simulink model "WDS2"  (R2022b)
settings: Solver=VariableStepAuto  StartTime=0.0  StopTime=86400  RelTol=0.034
libraries: sh_lib x46, nesl_utility x16, fl_lib x12, SignalEditorBlockLib x3
(part 1 of 2)
settings Model: Creator=philip  LastModifiedBy=philip
settings SolverCC: MaxConsecutiveMinStep=2

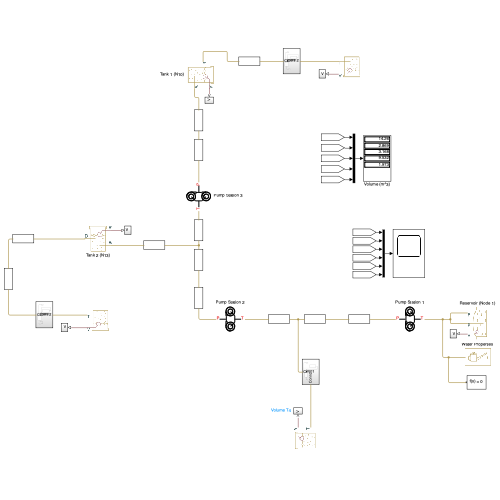
[thumbnail: Simulink's stored preview of the top-level diagram]
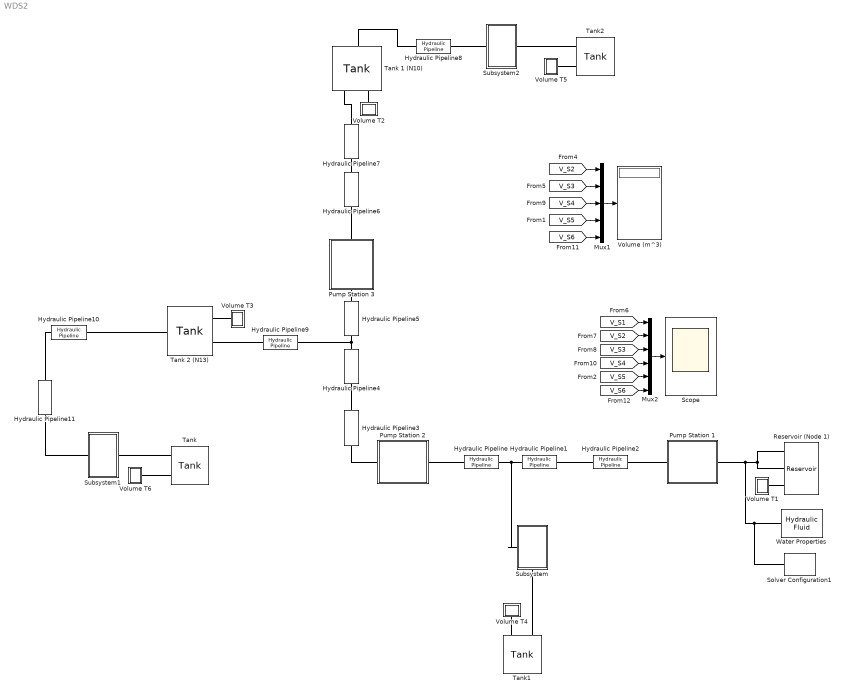
== system WDS2 ==
  Hydraulic Pipeline{,1..11} (12 alike) : sh_lib/Pipelines/Hydraulic Pipeline  cs_type=foundation.enum.pipeCrossSection.circular  d_in=0.01 m  area=1e-4 m^2  D_h=1.12e-2 m  s_factor=64  length=5 m  length_ad=1 m  roughness=15e-6 m  Re_lam=2000  Re_turb=4000  wall_type=foundation.enum.chamber_spec.rigid  pr_r_coef=2e-12 m/Pa  time_const=0.01 s  k_sh=1.4  initial_pressure=0 Pa
      settings: InternalSimscapePortConfiguration="{\"Bottom\":[],\"Left\":[{\"id\":\"A\",\"label\":\"A\",\"type\":\"foundation.hydraulic.hydraulic\"}],\"Right\":[{\"id\":\"B\",\"label\":\"B\",\"type\":\"foundation.hydraulic.hydraulic\"}],\"Top\":[]}"
  Mux1 : Mux  Inputs=5
  Mux2 : Mux  Inputs=6
  Pump Station 1 : Subsystem  Tag=PublishSubsystem
      mask Display:
      | plot(sin(0:0.5:4.5*pi)*0.9, cos(0:0.5:4.5*pi)*0.9+1.5)
      | plot(sin(0:0.5:4.5*pi)*0.5, cos(0:0.5:4.5*pi)*0.5+1.5)
      | plot(sin(0:0.5:4.5*pi)*0.9, cos(0:0.5:4.5*pi)*0.9-1.5)
      | plot(sin(0:0.5:4.5*pi)*0.5, cos(0:0.5:4.5*pi)*0.5-1.5)
      | 
      | plot([0 -0.9],[1.5 1.5-0.9])
      | plot([0 -0.9],[1.5 1.5-0.9]*-1)
      | 
      | plot([0.45 0.45 0.325 0.325]*2,[1.5 1.5-1.0 1.5-1.0 1.5-0.55])
      | plot([0.45 0.45 0.325 0.325]*2,[1.5 1.5-0.9 1.5-0.9 1.5-0.55]*-1)
      | 
      | plot([2.2 0.95]*-1,[0 0])
      | plot([2.2 0.95],[0 0])
      | 
      | plot([0.95 0.95]*-1,[-0.6 0.6])
      | plot([0.8 0.8],[-0.55 0.55])
      | 
      | 
      | color('white');plot(-3,-2.5);plot(3,2.5);
      | color('red');
      | port_label('LConn',1,'T');
      | port_label('RConn',1,'P');
  Pump Station 2 : Subsystem  Tag=PublishSubsystem
      mask Display:
      | plot(sin(0:0.5:4.5*pi)*0.9, cos(0:0.5:4.5*pi)*0.9+1.5)
      | plot(sin(0:0.5:4.5*pi)*0.5, cos(0:0.5:4.5*pi)*0.5+1.5)
      | plot(sin(0:0.5:4.5*pi)*0.9, cos(0:0.5:4.5*pi)*0.9-1.5)
      | plot(sin(0:0.5:4.5*pi)*0.5, cos(0:0.5:4.5*pi)*0.5-1.5)
      | 
      | plot([0 -0.9],[1.5 1.5-0.9])
      | plot([0 -0.9],[1.5 1.5-0.9]*-1)
      | 
      | plot([0.45 0.45 0.325 0.325]*2,[1.5 1.5-1.0 1.5-1.0 1.5-0.55])
      | plot([0.45 0.45 0.325 0.325]*2,[1.5 1.5-0.9 1.5-0.9 1.5-0.55]*-1)
      | 
      | plot([2.2 0.95]*-1,[0 0])
      | plot([2.2 0.95],[0 0])
      | 
      | plot([0.95 0.95]*-1,[-0.6 0.6])
      | plot([0.8 0.8],[-0.55 0.55])
      | 
      | 
      | color('white');plot(-3,-2.5);plot(3,2.5);
      | color('red');
      | port_label('LConn',1,'T');
      | port_label('RConn',1,'P');
  Pump Station 3 : Subsystem  Tag=PublishSubsystem
      mask Display:
      | plot(sin(0:0.5:4.5*pi)*0.9, cos(0:0.5:4.5*pi)*0.9+1.5)
      | plot(sin(0:0.5:4.5*pi)*0.5, cos(0:0.5:4.5*pi)*0.5+1.5)
      | plot(sin(0:0.5:4.5*pi)*0.9, cos(0:0.5:4.5*pi)*0.9-1.5)
      | plot(sin(0:0.5:4.5*pi)*0.5, cos(0:0.5:4.5*pi)*0.5-1.5)
      | 
      | plot([0 -0.9],[1.5 1.5-0.9])
      | plot([0 -0.9],[1.5 1.5-0.9]*-1)
      | 
      | plot([0.45 0.45 0.325 0.325]*2,[1.5 1.5-1.0 1.5-1.0 1.5-0.55])
      | plot([0.45 0.45 0.325 0.325]*2,[1.5 1.5-0.9 1.5-0.9 1.5-0.55]*-1)
      | 
      | plot([2.2 0.95]*-1,[0 0])
      | plot([2.2 0.95],[0 0])
      | 
      | plot([0.95 0.95]*-1,[-0.6 0.6])
      | plot([0.8 0.8],[-0.55 0.55])
      | 
      | 
      | color('white');plot(-3,-2.5);plot(3,2.5);
      | color('red');
      | port_label('LConn',1,'T');
      | port_label('RConn',1,'P');
  Reservoir (Node 1) : sh_lib/Hydraulic Utilities/Reservoir  press=0 Pa  init_volume=40 m^3  ret_diam=0.01 m  loss_coeff=1
      settings: InternalSimscapePortConfiguration="{\"Bottom\":[],\"Left\":[{\"id\":\"V\",\"label\":\"V\",\"type\":\"output\"},{\"id\":\"P\",\"label\":\"P\",\"type\":\"foundation.hydraulic.hydraulic\"},{\"id\":\"R\",\"label\":\"R\",\"type\":\"foundation.hydraulic.hydraulic\"}],\"Right\":[],\"Top\":[]}"
  Scope : Scope
  Solver Configuration1 : nesl_utility/Solver Configuration  PhysicalDomain=network_engine_domain  SubClassName=solver  LeftPortType=input  RightPortType=generic  Tones=[]  Harmonics=[]  SimulateNoise=off  Profile=off  UseLocalSampling=off  EnableSwitchedLinearOptims=on  FrequencyDomain=off  UseCCode=off  RelTol=0.001  AbsTol=1e-06  MinStep=1e-09  ToWorkspace=off  RevertToSquareIcSolve=off  NumHomotopyIterations=100  PhasorMode=off  PhasorModeNumHarmonics=1  ConsistencySolver=NEWTON_XTOL_AFTER_FTOL  IndexReductionMethod=DerivativeReplacement  DoDC=off  ResidualTolerance=1e-9  ConsistencyTolSource=GLOBAL  ConsistencyAbsTol=0.001  ConsistencyRelTol=0.001  ConsistencyTolFactor=0.034  UseLocalSolver=off  LocalSolverChoice=NE_BACKWARD_EULER_ADVANCER  ResolveIndetEquations=on  FunctionEvalNumThread=1  LocalSolverSampleTime=.001  DoFixedCost=off  MaxNonlinIter=3  MaxModeIter=2  ComputeImpulses=off  ImpulseIterations=2  LinearAlgebra=auto  LinearAlgebraNumThread=0  EquationFormulation=NE_TIME_EF  DelaysMemoryBudget=1024  AutomaticFiltering=on  FilteringTimeConstant=0.001  PartitionStorageMethod=AS_NEEDED  PartitionMemoryBudget=1024  PartitionMethod=FAST
  Subsystem : Subsystem
      settings: PortSchema="{\"entries\":[{\"content\":{\"sides\":[{\"content\":{\"connectorIds\":[\"LConn1\"]},\"type\":\"ConnectorPlacement.EquallySpacedRectSide\",\"uuid\":\"c5da6f35-8fa4-48b7-8a4a-4ae9db04ca9d\"},{\"content\":{\"connectorIds\":[],\"side\":\"RIGHT\"},\"type\":\"ConnectorPlacement.EquallySpacedRectSide\",\"uuid\":\"484dc1ab-2dc7-464f-80da-36af203a6e69\"},{\"content\":{\"connectorIds\":[],\"side\":\"TOP\"},\"type\":\"ConnectorPlacement.EquallySpacedRectSide\",\"uuid\":\"15bf6548-86e0-4373-a220-3fe0e1067d73\"},{\"content\":{\"connectorIds\":[\"RConn1\"],\"side\":\"BOTTOM\"},\"type\":\"ConnectorPlacement.EquallySpacedRectSide\",\"uuid\":\"b94051b1-e6bf-4793-98e6-5d6956093d36\"}]},\"type\":\"ConnectorPlacement.EquallySpacedConnector\",\"uuid\":\"b1159124-f196-4e4e-b402-5d78480e647c\"}],\"packageUris\":[\"http://schema.mathworks.com/mf0/Connector/R2020b\"],\"version\":\"1.0\"}"
  Subsystem1 : Subsystem
  Subsystem2 : Subsystem
  Tank : sh_lib/Low-Pressure Blocks/Tank  press=0 Pa  level_spec=1  tank_area=0.8 m^2  fluid_volume_tab=[0, .0028, .0065, .0114, .0176, .0252, .0344, .0436, .0512, .0574, .0623, .066, .0688, .0707, .072, .0727] m^3  fluid_level_tab=[0, .02, .04, .06, .08, .1, .12, .14, .16, .18, .2, .22, .24, .26, .28, .3] m  interp_method=1  extrap_method=1  pipe_diam=0.02 m  loss_coeff=1.2  g=9.80665 m/s^2  min_level=1e-3 m  fluid_level_check=0  volume_specify=off  volume_priority=High  volume=20 l  volume_nominal_specify=off  volume_nominal_unit=l  volume_nominal_value=1  level_specify=off  level_priority=None  level=0.025 m  level_nominal_specify=off  level_nominal_unit=m  level_nominal_value=1  pipe_diam_A=0.02 m  loss_coeff_A=1.2  height_B=0.8 m  pipe_diam_B=0.02 m  loss_coeff_B=1.2  height_C=0.8 m  pipe_diam_C=0.02 m  loss_coeff_C=1.2
      settings: InternalSimscapePortConfiguration="{\"Bottom\":[],\"Left\":[],\"Right\":[{\"id\":\"V\",\"label\":\"V\",\"type\":\"output\"},{\"id\":\"T\",\"label\":\"T\",\"type\":\"foundation.hydraulic.hydraulic\"}],\"Top\":[]}"
  Tank 1 (N10) : sh_lib/Low-Pressure Blocks/Tank  press=0 Pa  level_spec=1  tank_area=0.8 m^2  fluid_volume_tab=[0, .0028, .0065, .0114, .0176, .0252, .0344, .0436, .0512, .0574, .0623, .066, .0688, .0707, .072, .0727] m^3  fluid_level_tab=[0, .02, .04, .06, .08, .1, .12, .14, .16, .18, .2, .22, .24, .26, .28, .3] m  interp_method=1  extrap_method=1  pipe_diam=0.02 m  loss_coeff=1.2  g=9.80665 m/s^2  min_level=1e-3 m  fluid_level_check=0  volume_specify=off  volume_priority=High  volume=100 m^3  volume_nominal_specify=off  volume_nominal_unit=l  volume_nominal_value=1  level_specify=off  level_priority=None  level=station_3.fluid_level m  level_nominal_specify=off  level_nominal_unit=m  level_nominal_value=1  pipe_diam_A=0.01 m  loss_coeff_A=1.2  height_B=0.8 m  pipe_diam_B=0.01 m  loss_coeff_B=1.2  height_C=0.8 m  pipe_diam_C=0.02 m  loss_coeff_C=1.2
      settings: InternalSimscapePortConfiguration="{\"Bottom\":[],\"Left\":[{\"id\":\"B\",\"label\":\"B\",\"type\":\"foundation.hydraulic.hydraulic\"}],\"Right\":[{\"id\":\"V\",\"label\":\"V\",\"type\":\"output\"},{\"id\":\"A\",\"label\":\"A\",\"type\":\"foundation.hydraulic.hydraulic\"}],\"Top\":[]}"
  Tank 2 (N13) : sh_lib/Low-Pressure Blocks/Tank  press=0 Pa  level_spec=1  tank_area=0.8 m^2  fluid_volume_tab=[0, .0028, .0065, .0114, .0176, .0252, .0344, .0436, .0512, .0574, .0623, .066, .0688, .0707, .072, .0727] m^3  fluid_level_tab=[0, .02, .04, .06, .08, .1, .12, .14, .16, .18, .2, .22, .24, .26, .28, .3] m  interp_method=1  extrap_method=1  pipe_diam=0.02 m  loss_coeff=1.2  g=9.80665 m/s^2  min_level=1e-3 m  fluid_level_check=0  volume_specify=off  volume_priority=High  volume=100 m^3  volume_nominal_specify=off  volume_nominal_unit=l  volume_nominal_value=1  level_specify=off  level_priority=None  level=station_2.fluid_level m  level_nominal_specify=off  level_nominal_unit=m  level_nominal_value=1  pipe_diam_A=0.01 m  loss_coeff_A=1.2  height_B=0.8 m  pipe_diam_B=0.01 m  loss_coeff_B=1.2  height_C=0.8 m  pipe_diam_C=0.02 m  loss_coeff_C=1.2
      settings: InternalSimscapePortConfiguration="{\"Bottom\":[],\"Left\":[{\"id\":\"B\",\"label\":\"B\",\"type\":\"foundation.hydraulic.hydraulic\"}],\"Right\":[{\"id\":\"V\",\"label\":\"V\",\"type\":\"output\"},{\"id\":\"A\",\"label\":\"A\",\"type\":\"foundation.hydraulic.hydraulic\"}],\"Top\":[]}"
  Tank1 : sh_lib/Low-Pressure Blocks/Tank  press=0 Pa  level_spec=1  tank_area=0.8 m^2  fluid_volume_tab=[0, .0028, .0065, .0114, .0176, .0252, .0344, .0436, .0512, .0574, .0623, .066, .0688, .0707, .072, .0727] m^3  fluid_level_tab=[0, .02, .04, .06, .08, .1, .12, .14, .16, .18, .2, .22, .24, .26, .28, .3] m  interp_method=1  extrap_method=1  pipe_diam=0.02 m  loss_coeff=1.2  g=9.80665 m/s^2  min_level=1e-3 m  fluid_level_check=0  volume_specify=off  volume_priority=High  volume=20 l  volume_nominal_specify=off  volume_nominal_unit=l  volume_nominal_value=1  level_specify=off  level_priority=None  level=0.025 m  level_nominal_specify=off  level_nominal_unit=m  level_nominal_value=1  pipe_diam_A=0.02 m  loss_coeff_A=1.2  height_B=0.8 m  pipe_diam_B=0.02 m  loss_coeff_B=1.2  height_C=0.8 m  pipe_diam_C=0.02 m  loss_coeff_C=1.2
      settings: InternalSimscapePortConfiguration="{\"Bottom\":[],\"Left\":[],\"Right\":[{\"id\":\"V\",\"label\":\"V\",\"type\":\"output\"},{\"id\":\"T\",\"label\":\"T\",\"type\":\"foundation.hydraulic.hydraulic\"}],\"Top\":[]}"
  Tank2 : sh_lib/Low-Pressure Blocks/Tank  press=0 Pa  level_spec=1  tank_area=0.8 m^2  fluid_volume_tab=[0, .0028, .0065, .0114, .0176, .0252, .0344, .0436, .0512, .0574, .0623, .066, .0688, .0707, .072, .0727] m^3  fluid_level_tab=[0, .02, .04, .06, .08, .1, .12, .14, .16, .18, .2, .22, .24, .26, .28, .3] m  interp_method=1  extrap_method=1  pipe_diam=0.02 m  loss_coeff=1.2  g=9.80665 m/s^2  min_level=1e-3 m  fluid_level_check=0  volume_specify=off  volume_priority=High  volume=20 l  volume_nominal_specify=off  volume_nominal_unit=l  volume_nominal_value=1  level_specify=off  level_priority=None  level=0.025 m  level_nominal_specify=off  level_nominal_unit=m  level_nominal_value=1  pipe_diam_A=0.02 m  loss_coeff_A=1.2  height_B=0.8 m  pipe_diam_B=0.02 m  loss_coeff_B=1.2  height_C=0.8 m  pipe_diam_C=0.02 m  loss_coeff_C=1.2
      settings: InternalSimscapePortConfiguration="{\"Bottom\":[],\"Left\":[],\"Right\":[{\"id\":\"V\",\"label\":\"V\",\"type\":\"output\"},{\"id\":\"T\",\"label\":\"T\",\"type\":\"foundation.hydraulic.hydraulic\"}],\"Top\":[]}"
  Volume (m^3) : Display
  Volume T1 : Subsystem
  Volume T2 : Subsystem
  Volume T3 : Subsystem
  Volume T4 : Subsystem
  Volume T5 : Subsystem
  Volume T6 : Subsystem
  Water Properties : sh_lib/Hydraulic Utilities/Hydraulic Fluid  SelFluid=24  SysTemp=1  TrapAir=0.001  ViscDerFactor=1  range_error=2
  wires:
  Mux1/1 -> Volume (m^3)/1
  [V_S2] -> Mux1/1
  [V_S4] -> Mux1/3
  [V_S3] -> Mux1/2
  [V_S5] -> Mux1/4
  [V_S3] -> Mux2/3
  [V_S5] -> Mux2/5
  Mux2/1 -> Scope/1
  [V_S2] -> Mux2/2
  [V_S1] -> Mux2/1
  [V_S4] -> Mux2/4
  [V_S6] -> Mux1/5
  [V_S6] -> Mux2/6
  connections:
  Reservoir (Node 1)/LConn2 -- Pump Station 1/LConn1 -- Solver Configuration1/RConn1 -- Water Properties/RConn1 -- Reservoir (Node 1)/LConn3
  Hydraulic Pipeline2/RConn1 -- Hydraulic Pipeline1/LConn1
  Subsystem/LConn1 -- Hydraulic Pipeline1/RConn1 -- Hydraulic Pipeline/LConn1
  Hydraulic Pipeline4/LConn1 -- Hydraulic Pipeline3/RConn1
  Hydraulic Pipeline4/RConn1 -- Hydraulic Pipeline9/LConn1 -- Hydraulic Pipeline5/LConn1
  Hydraulic Pipeline7/LConn1 -- Hydraulic Pipeline6/RConn1
  Hydraulic Pipeline7/RConn1 -- Tank 1 (N10)/RConn2
  Hydraulic Pipeline8/LConn1 -- Tank 1 (N10)/LConn1
  Hydraulic Pipeline9/RConn1 -- Tank 2 (N13)/RConn2
  Hydraulic Pipeline11/LConn1 -- Hydraulic Pipeline10/RConn1
  Hydraulic Pipeline6/LConn1 -- Pump Station 3/RConn1
  Pump Station 3/LConn1 -- Hydraulic Pipeline5/RConn1
  Hydraulic Pipeline/RConn1 -- Pump Station 2/LConn1
  Pump Station 1/RConn1 -- Hydraulic Pipeline2/LConn1
  Volume T1/LConn1 -- Reservoir (Node 1)/LConn1
  Volume T2/LConn1 -- Tank 1 (N10)/RConn1
  Volume T3/LConn1 -- Tank 2 (N13)/RConn1
  Tank/RConn1 -- Volume T6/LConn1
  Tank1/RConn2 -- Subsystem/RConn1
  Tank1/RConn1 -- Volume T4/LConn1
  Hydraulic Pipeline8/RConn1 -- Subsystem2/LConn1
  Tank2/RConn1 -- Volume T5/LConn1
  Tank2/RConn2 -- Subsystem2/RConn1
  Hydraulic Pipeline10/LConn1 -- Tank 2 (N13)/LConn1
  Subsystem1/RConn1 -- Tank/RConn2
  Hydraulic Pipeline11/RConn1 -- Subsystem1/LConn1
  Pump Station 2/RConn1 -- Hydraulic Pipeline3/LConn1

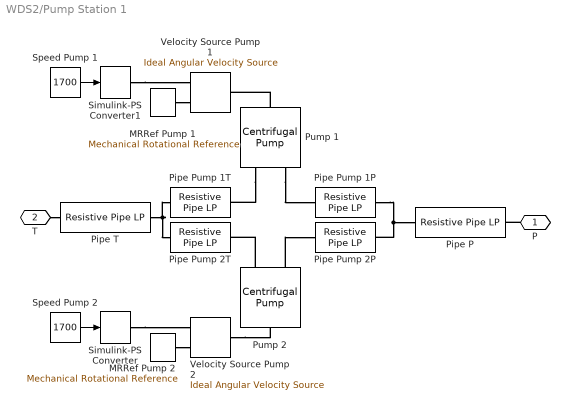
== system WDS2/Pump Station 1 ==
  MRRef Pump 1 : fl_lib/Mechanical/Rotational Elements/Mechanical Rotational Reference
  MRRef Pump 2 : fl_lib/Mechanical/Rotational Elements/Mechanical Rotational Reference
  Pipe P : sh_lib/Low-Pressure Blocks/Resistive Pipe LP  cs_type=1  d_in=station_1.pipe_diameter mm  area=1e-04 m^2  D_h=0.0112 m  s_factor=64  length=station_1.pipe_length_3 m  length_ad=1 m  roughness=0.005 mm  Re_lam=2e+03  Re_turb=4e+03  elevation_A=station_1.elevation m  elevation_B=station_1.elevation m  g=9.80665 m/s^2  pressure_drop_specify=off  pressure_drop_priority=None  pressure_drop=0 Pa  pressure_drop_nominal_specify=off  pressure_drop_nominal_unit=Pa  pressure_drop_nominal_value=1  flow_rate_specify=off  flow_rate_priority=None  flow_rate=0 m^3/s  flow_rate_nominal_specify=off  flow_rate_nominal_unit=m^3/s  flow_rate_nominal_value=1
      settings: InternalSimscapePortConfiguration="{\"Bottom\":[],\"Left\":[{\"id\":\"A\",\"label\":\"A\",\"type\":\"foundation.hydraulic.hydraulic\"}],\"Right\":[{\"id\":\"B\",\"label\":\"B\",\"type\":\"foundation.hydraulic.hydraulic\"}],\"Top\":[]}"
  Pipe Pump 1P : sh_lib/Low-Pressure Blocks/Resistive Pipe LP  cs_type=1  d_in=station_1.pipe_diameter mm  area=1e-04 m^2  D_h=0.0112 m  s_factor=64  length=station_1.pipe_length_2 m  length_ad=1 m  roughness=0.005 mm  Re_lam=2e+03  Re_turb=4e+03  elevation_A=station_1.elevation m  elevation_B=station_1.elevation m  g=9.80665 m/s^2  pressure_drop_specify=off  pressure_drop_priority=None  pressure_drop=0 Pa  pressure_drop_nominal_specify=off  pressure_drop_nominal_unit=Pa  pressure_drop_nominal_value=1  flow_rate_specify=off  flow_rate_priority=None  flow_rate=0 m^3/s  flow_rate_nominal_specify=off  flow_rate_nominal_unit=m^3/s  flow_rate_nominal_value=1
      settings: InternalSimscapePortConfiguration="{\"Bottom\":[],\"Left\":[{\"id\":\"A\",\"label\":\"A\",\"type\":\"foundation.hydraulic.hydraulic\"}],\"Right\":[{\"id\":\"B\",\"label\":\"B\",\"type\":\"foundation.hydraulic.hydraulic\"}],\"Top\":[]}"
  Pipe Pump 1T : sh_lib/Low-Pressure Blocks/Resistive Pipe LP  cs_type=1  d_in=station_1.pipe_diameter mm  area=1e-04 m^2  D_h=0.0112 m  s_factor=64  length=station_1.pipe_length_2 m  length_ad=1 m  roughness=0.005 mm  Re_lam=2e+03  Re_turb=4e+03  elevation_A=station_1.elevation m  elevation_B=station_1.elevation m  g=9.80665 m/s^2  pressure_drop_specify=off  pressure_drop_priority=None  pressure_drop=0 Pa  pressure_drop_nominal_specify=off  pressure_drop_nominal_unit=Pa  pressure_drop_nominal_value=1  flow_rate_specify=off  flow_rate_priority=None  flow_rate=0 m^3/s  flow_rate_nominal_specify=off  flow_rate_nominal_unit=m^3/s  flow_rate_nominal_value=1
      settings: InternalSimscapePortConfiguration="{\"Bottom\":[],\"Left\":[{\"id\":\"A\",\"label\":\"A\",\"type\":\"foundation.hydraulic.hydraulic\"}],\"Right\":[{\"id\":\"B\",\"label\":\"B\",\"type\":\"foundation.hydraulic.hydraulic\"}],\"Top\":[]}"
  Pipe Pump 2P : sh_lib/Low-Pressure Blocks/Resistive Pipe LP  cs_type=1  d_in=station_1.pipe_diameter mm  area=1e-04 m^2  D_h=0.0112 m  s_factor=64  length=station_1.pipe_length_2 m  length_ad=1 m  roughness=0.005 mm  Re_lam=2e+03  Re_turb=4e+03  elevation_A=station_1.elevation m  elevation_B=station_1.elevation m  g=9.80665 m/s^2  pressure_drop_specify=off  pressure_drop_priority=None  pressure_drop=0 Pa  pressure_drop_nominal_specify=off  pressure_drop_nominal_unit=Pa  pressure_drop_nominal_value=1  flow_rate_specify=off  flow_rate_priority=None  flow_rate=0 m^3/s  flow_rate_nominal_specify=off  flow_rate_nominal_unit=m^3/s  flow_rate_nominal_value=1
      settings: InternalSimscapePortConfiguration="{\"Bottom\":[],\"Left\":[{\"id\":\"A\",\"label\":\"A\",\"type\":\"foundation.hydraulic.hydraulic\"}],\"Right\":[{\"id\":\"B\",\"label\":\"B\",\"type\":\"foundation.hydraulic.hydraulic\"}],\"Top\":[]}"
  Pipe Pump 2T : sh_lib/Low-Pressure Blocks/Resistive Pipe LP  cs_type=1  d_in=station_1.pipe_diameter mm  area=1e-04 m^2  D_h=0.0112 m  s_factor=64  length=station_1.pipe_length_2 m  length_ad=1 m  roughness=0.005 mm  Re_lam=2e+03  Re_turb=4e+03  elevation_A=station_1.elevation m  elevation_B=station_1.elevation m  g=9.80665 m/s^2  pressure_drop_specify=off  pressure_drop_priority=None  pressure_drop=0 Pa  pressure_drop_nominal_specify=off  pressure_drop_nominal_unit=Pa  pressure_drop_nominal_value=1  flow_rate_specify=off  flow_rate_priority=None  flow_rate=0 m^3/s  flow_rate_nominal_specify=off  flow_rate_nominal_unit=m^3/s  flow_rate_nominal_value=1
      settings: InternalSimscapePortConfiguration="{\"Bottom\":[],\"Left\":[{\"id\":\"A\",\"label\":\"A\",\"type\":\"foundation.hydraulic.hydraulic\"}],\"Right\":[{\"id\":\"B\",\"label\":\"B\",\"type\":\"foundation.hydraulic.hydraulic\"}],\"Top\":[]}"
  Pipe T : sh_lib/Low-Pressure Blocks/Resistive Pipe LP  cs_type=1  d_in=station_1.pipe_diameter mm  area=1e-04 m^2  D_h=0.0112 m  s_factor=64  length=station_1.pipe_length_1 m  length_ad=1 m  roughness=0.005 mm  Re_lam=2e+03  Re_turb=4e+03  elevation_A=station_1.elevation m  elevation_B=station_1.elevation m  g=9.80665 m/s^2  pressure_drop_specify=off  pressure_drop_priority=None  pressure_drop=0 Pa  pressure_drop_nominal_specify=off  pressure_drop_nominal_unit=Pa  pressure_drop_nominal_value=1  flow_rate_specify=off  flow_rate_priority=None  flow_rate=0 m^3/s  flow_rate_nominal_specify=off  flow_rate_nominal_unit=m^3/s  flow_rate_nominal_value=1
      settings: InternalSimscapePortConfiguration="{\"Bottom\":[],\"Left\":[{\"id\":\"A\",\"label\":\"A\",\"type\":\"foundation.hydraulic.hydraulic\"}],\"Right\":[{\"id\":\"B\",\"label\":\"B\",\"type\":\"foundation.hydraulic.hydraulic\"}],\"Top\":[]}"
  Pump 1 : sh_lib/Pumps and Motors/Centrifugal Pump  mdl_type=2  c_1=326.8 Pa/(kg/m^3)  c_2=3.104e+04 Pa*s/kg  c_3=1.097e+07 Pa*s^2/(kg*m^3)  c_4=2.136e+05 Pa*s^2/(kg*m^3)  c_f=0.8  design_del=130 lpm  ref_velocity=1.77e+03 rpm  ref_density=1000 kg/m^3  leak_resistance=1e+8 Pa/(m^3/s)  T_const=0.1 N*m  trq_press_coeff=1e-6 N*m/Pa  pump_del_1D=pump_1.Q m^3/s  press_diff_1D=pump_1.P bar  pump_del_power_1D=pump_1.Q m^3/s  power_1D=pump_1.N W  pump_vel_2D="[  3.2e+03 3.3e+03 3.4e+03 3.5e+03 ] rpm"  pump_del_2D="[  0 50 100 150 200 250 300 350 ] lpm"  press_diff_2D="[  8.3 8.8 9.3 9.9 ; 7.8 8.3 8.8 9.4 ; 7.2 7.6 8.2 8.7 ; 6.5 7 7.5 8 ; 5.6 6.1 6.6 7.1 ; 4.7 5.2 5.7 6.2 ; 3.4 4 4.4 4.9 ; 2.3 2.7 3.4 3.6 ; ] bar"  pump_del_power_2D="[  0 50 100 150 200 250 300 350 ] lpm"  power_2D="[  1.223e+03 1.341e+03 1.467e+03 1.6e+03 ; 1.414e+03 1.551e+03 1.696e+03 1.85e+03 ; 1.636e+03 1.794e+03 1.962e+03 2.14e+03 ; 1.941e+03 2.129e+03 2.326e+03 2.54e+03 ; 2.224e+03 2.439e+03 2.66e+03 2.91e+03 ; 2.453e+03 2.691e+03 2.947e+03 3.21e+03 ; 2.757e+03 3.024e+03 3.307e+03 3.608e+03 ; 2.945e+03 3.23e+03 3.533e+03 3.854e+03 ; ] W"  omega_threshold=1e-9 rad/s  interp_method=2  extrap_method=1
      settings: InternalSimscapePortConfiguration="{\"Bottom\":[],\"Left\":[{\"id\":\"S\",\"label\":\"S\",\"type\":\"foundation.mechanical.rotational.rotational\"}],\"Right\":[{\"id\":\"P\",\"label\":\"P\",\"type\":\"foundation.hydraulic.hydraulic\"},{\"id\":\"T\",\"label\":\"T\",\"type\":\"foundation.hydraulic.hydraulic\"}],\"Top\":[]}"
  Pump 2 : sh_lib/Pumps and Motors/Centrifugal Pump  mdl_type=2  c_1=326.8 Pa/(kg/m^3)  c_2=3.104e+04 Pa*s/kg  c_3=1.097e+07 Pa*s^2/(kg*m^3)  c_4=2.136e+05 Pa*s^2/(kg*m^3)  c_f=0.8  design_del=130 lpm  ref_velocity=1.77e+03 rpm  ref_density=1000 kg/m^3  leak_resistance=1e+8 Pa/(m^3/s)  T_const=0.1 N*m  trq_press_coeff=1e-6 N*m/Pa  pump_del_1D=pump_1.Q m^3/s  press_diff_1D=pump_1.P bar  pump_del_power_1D=pump_1.Q m^3/s  power_1D=pump_1.N W  pump_vel_2D="[  3.2e+03 3.3e+03 3.4e+03 3.5e+03 ] rpm"  pump_del_2D="[  0 50 100 150 200 250 300 350 ] lpm"  press_diff_2D="[  8.3 8.8 9.3 9.9 ; 7.8 8.3 8.8 9.4 ; 7.2 7.6 8.2 8.7 ; 6.5 7 7.5 8 ; 5.6 6.1 6.6 7.1 ; 4.7 5.2 5.7 6.2 ; 3.4 4 4.4 4.9 ; 2.3 2.7 3.4 3.6 ; ] bar"  pump_del_power_2D="[  0 50 100 150 200 250 300 350 ] lpm"  power_2D="[  1.223e+03 1.341e+03 1.467e+03 1.6e+03 ; 1.414e+03 1.551e+03 1.696e+03 1.85e+03 ; 1.636e+03 1.794e+03 1.962e+03 2.14e+03 ; 1.941e+03 2.129e+03 2.326e+03 2.54e+03 ; 2.224e+03 2.439e+03 2.66e+03 2.91e+03 ; 2.453e+03 2.691e+03 2.947e+03 3.21e+03 ; 2.757e+03 3.024e+03 3.307e+03 3.608e+03 ; 2.945e+03 3.23e+03 3.533e+03 3.854e+03 ; ] W"  omega_threshold=1e-9 rad/s  interp_method=2  extrap_method=1
      settings: InternalSimscapePortConfiguration="{\"Bottom\":[],\"Left\":[{\"id\":\"S\",\"label\":\"S\",\"type\":\"foundation.mechanical.rotational.rotational\"}],\"Right\":[{\"id\":\"P\",\"label\":\"P\",\"type\":\"foundation.hydraulic.hydraulic\"},{\"id\":\"T\",\"label\":\"T\",\"type\":\"foundation.hydraulic.hydraulic\"}],\"Top\":[]}"
  Simulink-PS Converter : nesl_utility/Simulink-PS Converter  PhysicalDomain=network_engine_domain  SubClassName=ps_input  LeftPortType=input  RightPortType=output  PseudoPeriodic=off  Frequencies=[]  NoiseDistribution=none  NoiseParameters=[]  Unit=rpm  AffineConversion=off  FilteringAndDerivatives=zero  SimscapeFilterOrder=1  InputFilterTimeConstant=.001  UdotUserProvided=0
  Simulink-PS Converter1 : nesl_utility/Simulink-PS Converter  PhysicalDomain=network_engine_domain  SubClassName=ps_input  LeftPortType=input  RightPortType=output  PseudoPeriodic=off  Frequencies=[]  NoiseDistribution=none  NoiseParameters=[]  Unit=rpm  AffineConversion=off  FilteringAndDerivatives=zero  SimscapeFilterOrder=1  InputFilterTimeConstant=.001  UdotUserProvided=0
  Speed Pump 1 : Constant  Value=1700
  Speed Pump 2 : Constant  Value=1700
  Velocity Source Pump 1 : fl_lib/Mechanical/Mechanical Sources/Ideal Angular Velocity Source
  Velocity Source Pump 2 : fl_lib/Mechanical/Mechanical Sources/Ideal Angular Velocity Source
  P : PMIOPort  Side=Right
  T : PMIOPort  Port=2  Side=Left
  wires:
  Speed Pump 2/1 -> Simulink-PS Converter/1
  Speed Pump 1/1 -> Simulink-PS Converter1/1
  connections:
  Velocity Source Pump 2/LConn1 -- Pump 2/LConn1
  Pump 1/RConn1 -- Pipe Pump 1P/LConn1
  Pump 1/RConn2 -- Pipe Pump 1T/RConn1
  Pump 2/RConn2 -- Pipe Pump 2T/RConn1
  T/RConn1 -- Pipe T/LConn1
  Pump 2/RConn1 -- Pipe Pump 2P/LConn1
  Pipe T/RConn1 -- Pipe Pump 2T/LConn1 -- Pipe Pump 1T/LConn1
  Simulink-PS Converter/RConn1 -- Velocity Source Pump 2/RConn1
  MRRef Pump 2/LConn1 -- Velocity Source Pump 2/RConn2
  Pipe Pump 1P/RConn1 -- Pipe Pump 2P/RConn1 -- Pipe P/LConn1
  P/RConn1 -- Pipe P/RConn1
  MRRef Pump 1/LConn1 -- Velocity Source Pump 1/RConn2
  Pump 1/LConn1 -- Velocity Source Pump 1/LConn1
  Simulink-PS Converter1/RConn1 -- Velocity Source Pump 1/RConn1

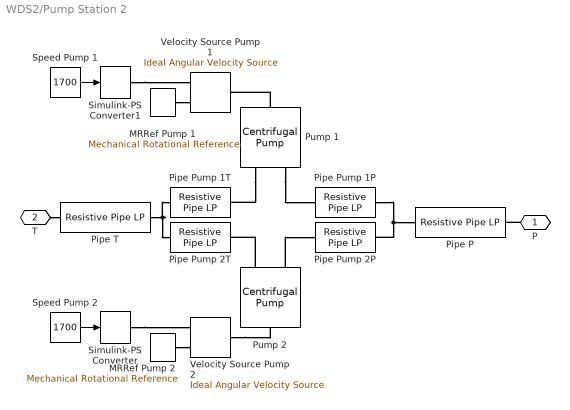
== system WDS2/Pump Station 2 ==
  MRRef Pump 1 : fl_lib/Mechanical/Rotational Elements/Mechanical Rotational Reference
  MRRef Pump 2 : fl_lib/Mechanical/Rotational Elements/Mechanical Rotational Reference
  Pipe P : sh_lib/Low-Pressure Blocks/Resistive Pipe LP  cs_type=1  d_in=station_1.pipe_diameter mm  area=1e-04 m^2  D_h=0.0112 m  s_factor=64  length=station_1.pipe_length_3 m  length_ad=1 m  roughness=0.005 mm  Re_lam=2e+03  Re_turb=4e+03  elevation_A=station_1.elevation m  elevation_B=station_1.elevation m  g=9.80665 m/s^2  pressure_drop_specify=off  pressure_drop_priority=None  pressure_drop=0 Pa  pressure_drop_nominal_specify=off  pressure_drop_nominal_unit=Pa  pressure_drop_nominal_value=1  flow_rate_specify=off  flow_rate_priority=None  flow_rate=0 m^3/s  flow_rate_nominal_specify=off  flow_rate_nominal_unit=m^3/s  flow_rate_nominal_value=1
      settings: InternalSimscapePortConfiguration="{\"Bottom\":[],\"Left\":[{\"id\":\"A\",\"label\":\"A\",\"type\":\"foundation.hydraulic.hydraulic\"}],\"Right\":[{\"id\":\"B\",\"label\":\"B\",\"type\":\"foundation.hydraulic.hydraulic\"}],\"Top\":[]}"
  Pipe Pump 1P : sh_lib/Low-Pressure Blocks/Resistive Pipe LP  cs_type=1  d_in=station_1.pipe_diameter mm  area=1e-04 m^2  D_h=0.0112 m  s_factor=64  length=station_1.pipe_length_2 m  length_ad=1 m  roughness=0.005 mm  Re_lam=2e+03  Re_turb=4e+03  elevation_A=station_1.elevation m  elevation_B=station_1.elevation m  g=9.80665 m/s^2  pressure_drop_specify=off  pressure_drop_priority=None  pressure_drop=0 Pa  pressure_drop_nominal_specify=off  pressure_drop_nominal_unit=Pa  pressure_drop_nominal_value=1  flow_rate_specify=off  flow_rate_priority=None  flow_rate=0 m^3/s  flow_rate_nominal_specify=off  flow_rate_nominal_unit=m^3/s  flow_rate_nominal_value=1
      settings: InternalSimscapePortConfiguration="{\"Bottom\":[],\"Left\":[{\"id\":\"A\",\"label\":\"A\",\"type\":\"foundation.hydraulic.hydraulic\"}],\"Right\":[{\"id\":\"B\",\"label\":\"B\",\"type\":\"foundation.hydraulic.hydraulic\"}],\"Top\":[]}"
  Pipe Pump 1T : sh_lib/Low-Pressure Blocks/Resistive Pipe LP  cs_type=1  d_in=station_1.pipe_diameter mm  area=1e-04 m^2  D_h=0.0112 m  s_factor=64  length=station_1.pipe_length_2 m  length_ad=1 m  roughness=0.005 mm  Re_lam=2e+03  Re_turb=4e+03  elevation_A=station_1.elevation m  elevation_B=station_1.elevation m  g=9.80665 m/s^2  pressure_drop_specify=off  pressure_drop_priority=None  pressure_drop=0 Pa  pressure_drop_nominal_specify=off  pressure_drop_nominal_unit=Pa  pressure_drop_nominal_value=1  flow_rate_specify=off  flow_rate_priority=None  flow_rate=0 m^3/s  flow_rate_nominal_specify=off  flow_rate_nominal_unit=m^3/s  flow_rate_nominal_value=1
      settings: InternalSimscapePortConfiguration="{\"Bottom\":[],\"Left\":[{\"id\":\"A\",\"label\":\"A\",\"type\":\"foundation.hydraulic.hydraulic\"}],\"Right\":[{\"id\":\"B\",\"label\":\"B\",\"type\":\"foundation.hydraulic.hydraulic\"}],\"Top\":[]}"
  Pipe Pump 2P : sh_lib/Low-Pressure Blocks/Resistive Pipe LP  cs_type=1  d_in=station_1.pipe_diameter mm  area=1e-04 m^2  D_h=0.0112 m  s_factor=64  length=station_1.pipe_length_2 m  length_ad=1 m  roughness=0.005 mm  Re_lam=2e+03  Re_turb=4e+03  elevation_A=station_1.elevation m  elevation_B=station_1.elevation m  g=9.80665 m/s^2  pressure_drop_specify=off  pressure_drop_priority=None  pressure_drop=0 Pa  pressure_drop_nominal_specify=off  pressure_drop_nominal_unit=Pa  pressure_drop_nominal_value=1  flow_rate_specify=off  flow_rate_priority=None  flow_rate=0 m^3/s  flow_rate_nominal_specify=off  flow_rate_nominal_unit=m^3/s  flow_rate_nominal_value=1
      settings: InternalSimscapePortConfiguration="{\"Bottom\":[],\"Left\":[{\"id\":\"A\",\"label\":\"A\",\"type\":\"foundation.hydraulic.hydraulic\"}],\"Right\":[{\"id\":\"B\",\"label\":\"B\",\"type\":\"foundation.hydraulic.hydraulic\"}],\"Top\":[]}"
  Pipe Pump 2T : sh_lib/Low-Pressure Blocks/Resistive Pipe LP  cs_type=1  d_in=station_1.pipe_diameter mm  area=1e-04 m^2  D_h=0.0112 m  s_factor=64  length=station_1.pipe_length_2 m  length_ad=1 m  roughness=0.005 mm  Re_lam=2e+03  Re_turb=4e+03  elevation_A=station_1.elevation m  elevation_B=station_1.elevation m  g=9.80665 m/s^2  pressure_drop_specify=off  pressure_drop_priority=None  pressure_drop=0 Pa  pressure_drop_nominal_specify=off  pressure_drop_nominal_unit=Pa  pressure_drop_nominal_value=1  flow_rate_specify=off  flow_rate_priority=None  flow_rate=0 m^3/s  flow_rate_nominal_specify=off  flow_rate_nominal_unit=m^3/s  flow_rate_nominal_value=1
      settings: InternalSimscapePortConfiguration="{\"Bottom\":[],\"Left\":[{\"id\":\"A\",\"label\":\"A\",\"type\":\"foundation.hydraulic.hydraulic\"}],\"Right\":[{\"id\":\"B\",\"label\":\"B\",\"type\":\"foundation.hydraulic.hydraulic\"}],\"Top\":[]}"
  Pipe T : sh_lib/Low-Pressure Blocks/Resistive Pipe LP  cs_type=1  d_in=station_1.pipe_diameter mm  area=1e-04 m^2  D_h=0.0112 m  s_factor=64  length=station_1.pipe_length_1 m  length_ad=1 m  roughness=0.005 mm  Re_lam=2e+03  Re_turb=4e+03  elevation_A=station_1.elevation m  elevation_B=station_1.elevation m  g=9.80665 m/s^2  pressure_drop_specify=off  pressure_drop_priority=None  pressure_drop=0 Pa  pressure_drop_nominal_specify=off  pressure_drop_nominal_unit=Pa  pressure_drop_nominal_value=1  flow_rate_specify=off  flow_rate_priority=None  flow_rate=0 m^3/s  flow_rate_nominal_specify=off  flow_rate_nominal_unit=m^3/s  flow_rate_nominal_value=1
      settings: InternalSimscapePortConfiguration="{\"Bottom\":[],\"Left\":[{\"id\":\"A\",\"label\":\"A\",\"type\":\"foundation.hydraulic.hydraulic\"}],\"Right\":[{\"id\":\"B\",\"label\":\"B\",\"type\":\"foundation.hydraulic.hydraulic\"}],\"Top\":[]}"
  Pump 1 : sh_lib/Pumps and Motors/Centrifugal Pump  mdl_type=2  c_1=326.8 Pa/(kg/m^3)  c_2=3.104e+04 Pa*s/kg  c_3=1.097e+07 Pa*s^2/(kg*m^3)  c_4=2.136e+05 Pa*s^2/(kg*m^3)  c_f=0.8  design_del=130 lpm  ref_velocity=1.77e+03 rpm  ref_density=1000 kg/m^3  leak_resistance=1e+8 Pa/(m^3/s)  T_const=0.1 N*m  trq_press_coeff=1e-6 N*m/Pa  pump_del_1D=pump_1.Q m^3/s  press_diff_1D=pump_1.P bar  pump_del_power_1D=pump_1.Q m^3/s  power_1D=pump_1.N W  pump_vel_2D="[  3.2e+03 3.3e+03 3.4e+03 3.5e+03 ] rpm"  pump_del_2D="[  0 50 100 150 200 250 300 350 ] lpm"  press_diff_2D="[  8.3 8.8 9.3 9.9 ; 7.8 8.3 8.8 9.4 ; 7.2 7.6 8.2 8.7 ; 6.5 7 7.5 8 ; 5.6 6.1 6.6 7.1 ; 4.7 5.2 5.7 6.2 ; 3.4 4 4.4 4.9 ; 2.3 2.7 3.4 3.6 ; ] bar"  pump_del_power_2D="[  0 50 100 150 200 250 300 350 ] lpm"  power_2D="[  1.223e+03 1.341e+03 1.467e+03 1.6e+03 ; 1.414e+03 1.551e+03 1.696e+03 1.85e+03 ; 1.636e+03 1.794e+03 1.962e+03 2.14e+03 ; 1.941e+03 2.129e+03 2.326e+03 2.54e+03 ; 2.224e+03 2.439e+03 2.66e+03 2.91e+03 ; 2.453e+03 2.691e+03 2.947e+03 3.21e+03 ; 2.757e+03 3.024e+03 3.307e+03 3.608e+03 ; 2.945e+03 3.23e+03 3.533e+03 3.854e+03 ; ] W"  omega_threshold=1e-9 rad/s  interp_method=2  extrap_method=1
      settings: InternalSimscapePortConfiguration="{\"Bottom\":[],\"Left\":[{\"id\":\"S\",\"label\":\"S\",\"type\":\"foundation.mechanical.rotational.rotational\"}],\"Right\":[{\"id\":\"P\",\"label\":\"P\",\"type\":\"foundation.hydraulic.hydraulic\"},{\"id\":\"T\",\"label\":\"T\",\"type\":\"foundation.hydraulic.hydraulic\"}],\"Top\":[]}"
  Pump 2 : sh_lib/Pumps and Motors/Centrifugal Pump  mdl_type=2  c_1=326.8 Pa/(kg/m^3)  c_2=3.104e+04 Pa*s/kg  c_3=1.097e+07 Pa*s^2/(kg*m^3)  c_4=2.136e+05 Pa*s^2/(kg*m^3)  c_f=0.8  design_del=130 lpm  ref_velocity=1.77e+03 rpm  ref_density=1000 kg/m^3  leak_resistance=1e+8 Pa/(m^3/s)  T_const=0.1 N*m  trq_press_coeff=1e-6 N*m/Pa  pump_del_1D=pump_1.Q m^3/s  press_diff_1D=pump_1.P bar  pump_del_power_1D=pump_1.Q m^3/s  power_1D=pump_1.N W  pump_vel_2D="[  3.2e+03 3.3e+03 3.4e+03 3.5e+03 ] rpm"  pump_del_2D="[  0 50 100 150 200 250 300 350 ] lpm"  press_diff_2D="[  8.3 8.8 9.3 9.9 ; 7.8 8.3 8.8 9.4 ; 7.2 7.6 8.2 8.7 ; 6.5 7 7.5 8 ; 5.6 6.1 6.6 7.1 ; 4.7 5.2 5.7 6.2 ; 3.4 4 4.4 4.9 ; 2.3 2.7 3.4 3.6 ; ] bar"  pump_del_power_2D="[  0 50 100 150 200 250 300 350 ] lpm"  power_2D="[  1.223e+03 1.341e+03 1.467e+03 1.6e+03 ; 1.414e+03 1.551e+03 1.696e+03 1.85e+03 ; 1.636e+03 1.794e+03 1.962e+03 2.14e+03 ; 1.941e+03 2.129e+03 2.326e+03 2.54e+03 ; 2.224e+03 2.439e+03 2.66e+03 2.91e+03 ; 2.453e+03 2.691e+03 2.947e+03 3.21e+03 ; 2.757e+03 3.024e+03 3.307e+03 3.608e+03 ; 2.945e+03 3.23e+03 3.533e+03 3.854e+03 ; ] W"  omega_threshold=1e-9 rad/s  interp_method=2  extrap_method=1
      settings: InternalSimscapePortConfiguration="{\"Bottom\":[],\"Left\":[{\"id\":\"S\",\"label\":\"S\",\"type\":\"foundation.mechanical.rotational.rotational\"}],\"Right\":[{\"id\":\"P\",\"label\":\"P\",\"type\":\"foundation.hydraulic.hydraulic\"},{\"id\":\"T\",\"label\":\"T\",\"type\":\"foundation.hydraulic.hydraulic\"}],\"Top\":[]}"
  Simulink-PS Converter : nesl_utility/Simulink-PS Converter  PhysicalDomain=network_engine_domain  SubClassName=ps_input  LeftPortType=input  RightPortType=output  PseudoPeriodic=off  Frequencies=[]  NoiseDistribution=none  NoiseParameters=[]  Unit=rpm  AffineConversion=off  FilteringAndDerivatives=zero  SimscapeFilterOrder=1  InputFilterTimeConstant=.001  UdotUserProvided=0
  Simulink-PS Converter1 : nesl_utility/Simulink-PS Converter  PhysicalDomain=network_engine_domain  SubClassName=ps_input  LeftPortType=input  RightPortType=output  PseudoPeriodic=off  Frequencies=[]  NoiseDistribution=none  NoiseParameters=[]  Unit=rpm  AffineConversion=off  FilteringAndDerivatives=zero  SimscapeFilterOrder=1  InputFilterTimeConstant=.001  UdotUserProvided=0
  Speed Pump 1 : Constant  Value=1700
  Speed Pump 2 : Constant  Value=1700
  Velocity Source Pump 1 : fl_lib/Mechanical/Mechanical Sources/Ideal Angular Velocity Source
  Velocity Source Pump 2 : fl_lib/Mechanical/Mechanical Sources/Ideal Angular Velocity Source
  P : PMIOPort  Side=Right
  T : PMIOPort  Port=2  Side=Left
  wires:
  Speed Pump 2/1 -> Simulink-PS Converter/1
  Speed Pump 1/1 -> Simulink-PS Converter1/1
  connections:
  Velocity Source Pump 2/LConn1 -- Pump 2/LConn1
  Pump 1/RConn1 -- Pipe Pump 1P/LConn1
  Pump 1/RConn2 -- Pipe Pump 1T/RConn1
  Pump 2/RConn2 -- Pipe Pump 2T/RConn1
  T/RConn1 -- Pipe T/LConn1
  Pump 2/RConn1 -- Pipe Pump 2P/LConn1
  Pipe T/RConn1 -- Pipe Pump 2T/LConn1 -- Pipe Pump 1T/LConn1
  Simulink-PS Converter/RConn1 -- Velocity Source Pump 2/RConn1
  MRRef Pump 2/LConn1 -- Velocity Source Pump 2/RConn2
  Pipe Pump 1P/RConn1 -- Pipe Pump 2P/RConn1 -- Pipe P/LConn1
  P/RConn1 -- Pipe P/RConn1
  MRRef Pump 1/LConn1 -- Velocity Source Pump 1/RConn2
  Pump 1/LConn1 -- Velocity Source Pump 1/LConn1
  Simulink-PS Converter1/RConn1 -- Velocity Source Pump 1/RConn1

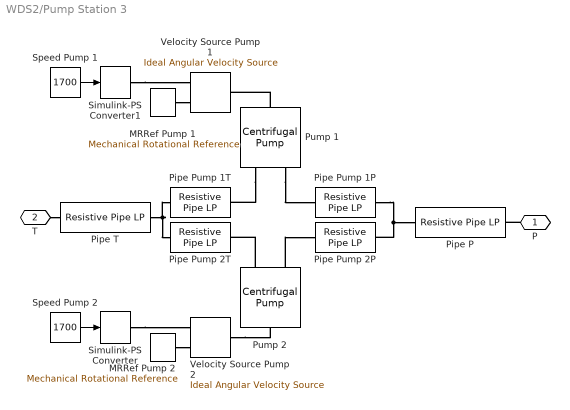
== system WDS2/Pump Station 3 ==
  MRRef Pump 1 : fl_lib/Mechanical/Rotational Elements/Mechanical Rotational Reference
  MRRef Pump 2 : fl_lib/Mechanical/Rotational Elements/Mechanical Rotational Reference
  Pipe P : sh_lib/Low-Pressure Blocks/Resistive Pipe LP  cs_type=1  d_in=station_1.pipe_diameter mm  area=1e-04 m^2  D_h=0.0112 m  s_factor=64  length=station_1.pipe_length_3 m  length_ad=1 m  roughness=0.005 mm  Re_lam=2e+03  Re_turb=4e+03  elevation_A=station_1.elevation m  elevation_B=station_1.elevation m  g=9.80665 m/s^2  pressure_drop_specify=off  pressure_drop_priority=None  pressure_drop=0 Pa  pressure_drop_nominal_specify=off  pressure_drop_nominal_unit=Pa  pressure_drop_nominal_value=1  flow_rate_specify=off  flow_rate_priority=None  flow_rate=0 m^3/s  flow_rate_nominal_specify=off  flow_rate_nominal_unit=m^3/s  flow_rate_nominal_value=1
      settings: InternalSimscapePortConfiguration="{\"Bottom\":[],\"Left\":[{\"id\":\"A\",\"label\":\"A\",\"type\":\"foundation.hydraulic.hydraulic\"}],\"Right\":[{\"id\":\"B\",\"label\":\"B\",\"type\":\"foundation.hydraulic.hydraulic\"}],\"Top\":[]}"
  Pipe Pump 1P : sh_lib/Low-Pressure Blocks/Resistive Pipe LP  cs_type=1  d_in=station_1.pipe_diameter mm  area=1e-04 m^2  D_h=0.0112 m  s_factor=64  length=station_1.pipe_length_2 m  length_ad=1 m  roughness=0.005 mm  Re_lam=2e+03  Re_turb=4e+03  elevation_A=station_1.elevation m  elevation_B=station_1.elevation m  g=9.80665 m/s^2  pressure_drop_specify=off  pressure_drop_priority=None  pressure_drop=0 Pa  pressure_drop_nominal_specify=off  pressure_drop_nominal_unit=Pa  pressure_drop_nominal_value=1  flow_rate_specify=off  flow_rate_priority=None  flow_rate=0 m^3/s  flow_rate_nominal_specify=off  flow_rate_nominal_unit=m^3/s  flow_rate_nominal_value=1
      settings: InternalSimscapePortConfiguration="{\"Bottom\":[],\"Left\":[{\"id\":\"A\",\"label\":\"A\",\"type\":\"foundation.hydraulic.hydraulic\"}],\"Right\":[{\"id\":\"B\",\"label\":\"B\",\"type\":\"foundation.hydraulic.hydraulic\"}],\"Top\":[]}"
  Pipe Pump 1T : sh_lib/Low-Pressure Blocks/Resistive Pipe LP  cs_type=1  d_in=station_1.pipe_diameter mm  area=1e-04 m^2  D_h=0.0112 m  s_factor=64  length=station_1.pipe_length_2 m  length_ad=1 m  roughness=0.005 mm  Re_lam=2e+03  Re_turb=4e+03  elevation_A=station_1.elevation m  elevation_B=station_1.elevation m  g=9.80665 m/s^2  pressure_drop_specify=off  pressure_drop_priority=None  pressure_drop=0 Pa  pressure_drop_nominal_specify=off  pressure_drop_nominal_unit=Pa  pressure_drop_nominal_value=1  flow_rate_specify=off  flow_rate_priority=None  flow_rate=0 m^3/s  flow_rate_nominal_specify=off  flow_rate_nominal_unit=m^3/s  flow_rate_nominal_value=1
      settings: InternalSimscapePortConfiguration="{\"Bottom\":[],\"Left\":[{\"id\":\"A\",\"label\":\"A\",\"type\":\"foundation.hydraulic.hydraulic\"}],\"Right\":[{\"id\":\"B\",\"label\":\"B\",\"type\":\"foundation.hydraulic.hydraulic\"}],\"Top\":[]}"
  Pipe Pump 2P : sh_lib/Low-Pressure Blocks/Resistive Pipe LP  cs_type=1  d_in=station_1.pipe_diameter mm  area=1e-04 m^2  D_h=0.0112 m  s_factor=64  length=station_1.pipe_length_2 m  length_ad=1 m  roughness=0.005 mm  Re_lam=2e+03  Re_turb=4e+03  elevation_A=station_1.elevation m  elevation_B=station_1.elevation m  g=9.80665 m/s^2  pressure_drop_specify=off  pressure_drop_priority=None  pressure_drop=0 Pa  pressure_drop_nominal_specify=off  pressure_drop_nominal_unit=Pa  pressure_drop_nominal_value=1  flow_rate_specify=off  flow_rate_priority=None  flow_rate=0 m^3/s  flow_rate_nominal_specify=off  flow_rate_nominal_unit=m^3/s  flow_rate_nominal_value=1
      settings: InternalSimscapePortConfiguration="{\"Bottom\":[],\"Left\":[{\"id\":\"A\",\"label\":\"A\",\"type\":\"foundation.hydraulic.hydraulic\"}],\"Right\":[{\"id\":\"B\",\"label\":\"B\",\"type\":\"foundation.hydraulic.hydraulic\"}],\"Top\":[]}"
  Pipe Pump 2T : sh_lib/Low-Pressure Blocks/Resistive Pipe LP  cs_type=1  d_in=station_1.pipe_diameter mm  area=1e-04 m^2  D_h=0.0112 m  s_factor=64  length=station_1.pipe_length_2 m  length_ad=1 m  roughness=0.005 mm  Re_lam=2e+03  Re_turb=4e+03  elevation_A=station_1.elevation m  elevation_B=station_1.elevation m  g=9.80665 m/s^2  pressure_drop_specify=off  pressure_drop_priority=None  pressure_drop=0 Pa  pressure_drop_nominal_specify=off  pressure_drop_nominal_unit=Pa  pressure_drop_nominal_value=1  flow_rate_specify=off  flow_rate_priority=None  flow_rate=0 m^3/s  flow_rate_nominal_specify=off  flow_rate_nominal_unit=m^3/s  flow_rate_nominal_value=1
      settings: InternalSimscapePortConfiguration="{\"Bottom\":[],\"Left\":[{\"id\":\"A\",\"label\":\"A\",\"type\":\"foundation.hydraulic.hydraulic\"}],\"Right\":[{\"id\":\"B\",\"label\":\"B\",\"type\":\"foundation.hydraulic.hydraulic\"}],\"Top\":[]}"
  Pipe T : sh_lib/Low-Pressure Blocks/Resistive Pipe LP  cs_type=1  d_in=station_1.pipe_diameter mm  area=1e-04 m^2  D_h=0.0112 m  s_factor=64  length=station_1.pipe_length_1 m  length_ad=1 m  roughness=0.005 mm  Re_lam=2e+03  Re_turb=4e+03  elevation_A=station_1.elevation m  elevation_B=station_1.elevation m  g=9.80665 m/s^2  pressure_drop_specify=off  pressure_drop_priority=None  pressure_drop=0 Pa  pressure_drop_nominal_specify=off  pressure_drop_nominal_unit=Pa  pressure_drop_nominal_value=1  flow_rate_specify=off  flow_rate_priority=None  flow_rate=0 m^3/s  flow_rate_nominal_specify=off  flow_rate_nominal_unit=m^3/s  flow_rate_nominal_value=1
      settings: InternalSimscapePortConfiguration="{\"Bottom\":[],\"Left\":[{\"id\":\"A\",\"label\":\"A\",\"type\":\"foundation.hydraulic.hydraulic\"}],\"Right\":[{\"id\":\"B\",\"label\":\"B\",\"type\":\"foundation.hydraulic.hydraulic\"}],\"Top\":[]}"
  Pump 1 : sh_lib/Pumps and Motors/Centrifugal Pump  mdl_type=2  c_1=326.8 Pa/(kg/m^3)  c_2=3.104e+04 Pa*s/kg  c_3=1.097e+07 Pa*s^2/(kg*m^3)  c_4=2.136e+05 Pa*s^2/(kg*m^3)  c_f=0.8  design_del=130 lpm  ref_velocity=1.77e+03 rpm  ref_density=1000 kg/m^3  leak_resistance=1e+8 Pa/(m^3/s)  T_const=0.1 N*m  trq_press_coeff=1e-6 N*m/Pa  pump_del_1D=pump_1.Q m^3/s  press_diff_1D=pump_1.P bar  pump_del_power_1D=pump_1.Q m^3/s  power_1D=pump_1.N W  pump_vel_2D="[  3.2e+03 3.3e+03 3.4e+03 3.5e+03 ] rpm"  pump_del_2D="[  0 50 100 150 200 250 300 350 ] lpm"  press_diff_2D="[  8.3 8.8 9.3 9.9 ; 7.8 8.3 8.8 9.4 ; 7.2 7.6 8.2 8.7 ; 6.5 7 7.5 8 ; 5.6 6.1 6.6 7.1 ; 4.7 5.2 5.7 6.2 ; 3.4 4 4.4 4.9 ; 2.3 2.7 3.4 3.6 ; ] bar"  pump_del_power_2D="[  0 50 100 150 200 250 300 350 ] lpm"  power_2D="[  1.223e+03 1.341e+03 1.467e+03 1.6e+03 ; 1.414e+03 1.551e+03 1.696e+03 1.85e+03 ; 1.636e+03 1.794e+03 1.962e+03 2.14e+03 ; 1.941e+03 2.129e+03 2.326e+03 2.54e+03 ; 2.224e+03 2.439e+03 2.66e+03 2.91e+03 ; 2.453e+03 2.691e+03 2.947e+03 3.21e+03 ; 2.757e+03 3.024e+03 3.307e+03 3.608e+03 ; 2.945e+03 3.23e+03 3.533e+03 3.854e+03 ; ] W"  omega_threshold=1e-9 rad/s  interp_method=2  extrap_method=1
      settings: InternalSimscapePortConfiguration="{\"Bottom\":[],\"Left\":[{\"id\":\"S\",\"label\":\"S\",\"type\":\"foundation.mechanical.rotational.rotational\"}],\"Right\":[{\"id\":\"P\",\"label\":\"P\",\"type\":\"foundation.hydraulic.hydraulic\"},{\"id\":\"T\",\"label\":\"T\",\"type\":\"foundation.hydraulic.hydraulic\"}],\"Top\":[]}"
  Pump 2 : sh_lib/Pumps and Motors/Centrifugal Pump  mdl_type=2  c_1=326.8 Pa/(kg/m^3)  c_2=3.104e+04 Pa*s/kg  c_3=1.097e+07 Pa*s^2/(kg*m^3)  c_4=2.136e+05 Pa*s^2/(kg*m^3)  c_f=0.8  design_del=130 lpm  ref_velocity=1.77e+03 rpm  ref_density=1000 kg/m^3  leak_resistance=1e+8 Pa/(m^3/s)  T_const=0.1 N*m  trq_press_coeff=1e-6 N*m/Pa  pump_del_1D=pump_1.Q m^3/s  press_diff_1D=pump_1.P bar  pump_del_power_1D=pump_1.Q m^3/s  power_1D=pump_1.N W  pump_vel_2D="[  3.2e+03 3.3e+03 3.4e+03 3.5e+03 ] rpm"  pump_del_2D="[  0 50 100 150 200 250 300 350 ] lpm"  press_diff_2D="[  8.3 8.8 9.3 9.9 ; 7.8 8.3 8.8 9.4 ; 7.2 7.6 8.2 8.7 ; 6.5 7 7.5 8 ; 5.6 6.1 6.6 7.1 ; 4.7 5.2 5.7 6.2 ; 3.4 4 4.4 4.9 ; 2.3 2.7 3.4 3.6 ; ] bar"  pump_del_power_2D="[  0 50 100 150 200 250 300 350 ] lpm"  power_2D="[  1.223e+03 1.341e+03 1.467e+03 1.6e+03 ; 1.414e+03 1.551e+03 1.696e+03 1.85e+03 ; 1.636e+03 1.794e+03 1.962e+03 2.14e+03 ; 1.941e+03 2.129e+03 2.326e+03 2.54e+03 ; 2.224e+03 2.439e+03 2.66e+03 2.91e+03 ; 2.453e+03 2.691e+03 2.947e+03 3.21e+03 ; 2.757e+03 3.024e+03 3.307e+03 3.608e+03 ; 2.945e+03 3.23e+03 3.533e+03 3.854e+03 ; ] W"  omega_threshold=1e-9 rad/s  interp_method=2  extrap_method=1
      settings: InternalSimscapePortConfiguration="{\"Bottom\":[],\"Left\":[{\"id\":\"S\",\"label\":\"S\",\"type\":\"foundation.mechanical.rotational.rotational\"}],\"Right\":[{\"id\":\"P\",\"label\":\"P\",\"type\":\"foundation.hydraulic.hydraulic\"},{\"id\":\"T\",\"label\":\"T\",\"type\":\"foundation.hydraulic.hydraulic\"}],\"Top\":[]}"
  Simulink-PS Converter : nesl_utility/Simulink-PS Converter  PhysicalDomain=network_engine_domain  SubClassName=ps_input  LeftPortType=input  RightPortType=output  PseudoPeriodic=off  Frequencies=[]  NoiseDistribution=none  NoiseParameters=[]  Unit=rpm  AffineConversion=off  FilteringAndDerivatives=zero  SimscapeFilterOrder=1  InputFilterTimeConstant=.001  UdotUserProvided=0
  Simulink-PS Converter1 : nesl_utility/Simulink-PS Converter  PhysicalDomain=network_engine_domain  SubClassName=ps_input  LeftPortType=input  RightPortType=output  PseudoPeriodic=off  Frequencies=[]  NoiseDistribution=none  NoiseParameters=[]  Unit=rpm  AffineConversion=off  FilteringAndDerivatives=zero  SimscapeFilterOrder=1  InputFilterTimeConstant=.001  UdotUserProvided=0
  Speed Pump 1 : Constant  Value=1700
  Speed Pump 2 : Constant  Value=1700
  Velocity Source Pump 1 : fl_lib/Mechanical/Mechanical Sources/Ideal Angular Velocity Source
  Velocity Source Pump 2 : fl_lib/Mechanical/Mechanical Sources/Ideal Angular Velocity Source
  P : PMIOPort  Side=Right
  T : PMIOPort  Port=2  Side=Left
  wires:
  Speed Pump 2/1 -> Simulink-PS Converter/1
  Speed Pump 1/1 -> Simulink-PS Converter1/1
  connections:
  Velocity Source Pump 2/LConn1 -- Pump 2/LConn1
  Pump 1/RConn1 -- Pipe Pump 1P/LConn1
  Pump 1/RConn2 -- Pipe Pump 1T/RConn1
  Pump 2/RConn2 -- Pipe Pump 2T/RConn1
  T/RConn1 -- Pipe T/LConn1
  Pump 2/RConn1 -- Pipe Pump 2P/LConn1
  Pipe T/RConn1 -- Pipe Pump 2T/LConn1 -- Pipe Pump 1T/LConn1
  Simulink-PS Converter/RConn1 -- Velocity Source Pump 2/RConn1
  MRRef Pump 2/LConn1 -- Velocity Source Pump 2/RConn2
  Pipe Pump 1P/RConn1 -- Pipe Pump 2P/RConn1 -- Pipe P/LConn1
  P/RConn1 -- Pipe P/RConn1
  MRRef Pump 1/LConn1 -- Velocity Source Pump 1/RConn2
  Pump 1/LConn1 -- Velocity Source Pump 1/LConn1
  Simulink-PS Converter1/RConn1 -- Velocity Source Pump 1/RConn1

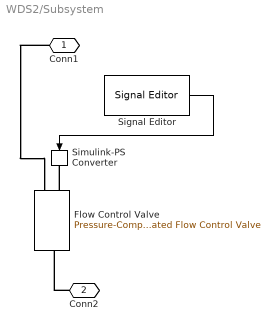
== system WDS2/Subsystem ==
  Flow Control Valve : sh_lib/Valves/Flow Control Valves/Pressure-Compensated Flow Control Valve  Tag=Factory Generic  mdl_type=1  area_max=0.86e-4 m^2  opening_max=0.016 m  opening_tab="[  -0.002 0 0.005 0.015 ] m"  area_tab="[  1e-12 4e-12 1e-05 1.02e-05 ] m^2"  interp_method=1  extrap_method=1  pr_dif=6e+05 Pa  reg_range=5e+04 Pa  C_d=0.7  x_0=0 m  A_leak=1e-12 m^2  lam_spec=1  B_lam=0.999  Re_cr=12
      settings: InternalSimscapePortConfiguration="{\"Bottom\":[],\"Left\":[{\"id\":\"C\",\"label\":\"C\",\"type\":\"input\"},{\"id\":\"A\",\"label\":\"A\",\"type\":\"foundation.hydraulic.hydraulic\"}],\"Right\":[{\"id\":\"B\",\"label\":\"B\",\"type\":\"foundation.hydraulic.hydraulic\"}],\"Top\":[]}"
  Signal Editor : SignalEditorBlockLib/Signal Editor  FileName=/Users/philip/Desktop/untitled folder/Untitled.mat  ActiveScenario=Scenario  ActiveSignal=Signal 1  IsBus=off  OutputBusObjectStr=Bus: BusObject  SampleTime=0  Interpolate=off  ZeroCross=off  OutputAfterFinalValue=Setting to zero  Unit=inherit  PreserveSignalName=on
  Simulink-PS Converter : nesl_utility/Simulink-PS Converter  PhysicalDomain=network_engine_domain  SubClassName=ps_input  LeftPortType=input  RightPortType=output  PseudoPeriodic=off  Frequencies=[]  NoiseDistribution=none  NoiseParameters=[]  Unit=1  AffineConversion=off  FilteringAndDerivatives=provide  SimscapeFilterOrder=1  InputFilterTimeConstant=0.001  UdotUserProvided=0
  Conn1 : PMIOPort  Side=Left
  Conn2 : PMIOPort  Port=2  Side=Right
  wires:
  Signal Editor/1 -> Simulink-PS Converter/1
  connections:
  Conn1/RConn1 -- Flow Control Valve/LConn2
  Conn2/RConn1 -- Flow Control Valve/RConn1
  Flow Control Valve/LConn1 -- Simulink-PS Converter/RConn1

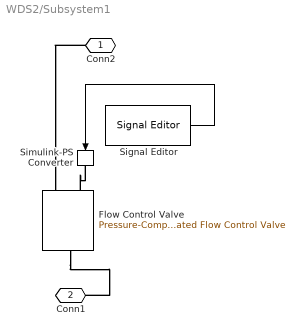
== system WDS2/Subsystem1 ==
  Flow Control Valve : sh_lib/Valves/Flow Control Valves/Pressure-Compensated Flow Control Valve  Tag=Factory Generic  mdl_type=1  area_max=0.86e-4 m^2  opening_max=0.016 m  opening_tab="[  -0.002 0 0.005 0.015 ] m"  area_tab="[  1e-12 4e-12 1e-05 1.02e-05 ] m^2"  interp_method=1  extrap_method=1  pr_dif=6e+05 Pa  reg_range=5e+04 Pa  C_d=0.7  x_0=0 m  A_leak=1e-12 m^2  lam_spec=1  B_lam=0.999  Re_cr=12
      settings: InternalSimscapePortConfiguration="{\"Bottom\":[],\"Left\":[{\"id\":\"C\",\"label\":\"C\",\"type\":\"input\"},{\"id\":\"A\",\"label\":\"A\",\"type\":\"foundation.hydraulic.hydraulic\"}],\"Right\":[{\"id\":\"B\",\"label\":\"B\",\"type\":\"foundation.hydraulic.hydraulic\"}],\"Top\":[]}"
  Signal Editor : SignalEditorBlockLib/Signal Editor  FileName=/Users/philip/Desktop/untitled folder/Untitled.mat  ActiveScenario=Scenario  ActiveSignal=Signal 1  IsBus=off  OutputBusObjectStr=Bus: BusObject  SampleTime=0  Interpolate=off  ZeroCross=off  OutputAfterFinalValue=Setting to zero  Unit=inherit  PreserveSignalName=on
  Simulink-PS Converter : nesl_utility/Simulink-PS Converter  PhysicalDomain=network_engine_domain  SubClassName=ps_input  LeftPortType=input  RightPortType=output  PseudoPeriodic=off  Frequencies=[]  NoiseDistribution=none  NoiseParameters=[]  Unit=1  AffineConversion=off  FilteringAndDerivatives=provide  SimscapeFilterOrder=1  InputFilterTimeConstant=0.001  UdotUserProvided=0
  Conn2 : PMIOPort  Side=Right
  Conn1 : PMIOPort  Port=2  Side=Left
  wires:
  Signal Editor/1 -> Simulink-PS Converter/1
  connections:
  Conn2/RConn1 -- Flow Control Valve/LConn2
  Flow Control Valve/LConn1 -- Simulink-PS Converter/RConn1
  Flow Control Valve/RConn1 -- Conn1/RConn1
